simulink model "discrete_ex"  (R2024a)
settings: Solver=ode15s  StartTime=0.0  StopTime=.2  FixedStep=T/50  RelTol=1e-3
undefined symbols (not defined in the file): Down, T, Up, Vo_ref
libraries: fl_lib x10, nesl_utility x10, ee_lib x2, simulink x1, eePwmGenerator x1
settings Model: Creator=guerr  LastModifiedBy=nicholas
settings SolverCC: ZeroCrossAlgorithm=Adaptive  AlgebraicLoopSolver=LineSearch
settings DebuggingCC: IgnoredZcDiagnostic=none  UnconnectedInputMsg=warning  UnconnectedOutputMsg=warning  UnconnectedLineMsg=warning
settings ModelReferenceCC: EnableRefExpFcnMdlSchedulingChecks=on
settings SFSimCC: CustomCodeUndefinedFunction=UseInterfaceOnly
settings RTWCC: GPUComputeCapability=3.5
settings SimscapeCC: SimscapeNormalizeSystem=off

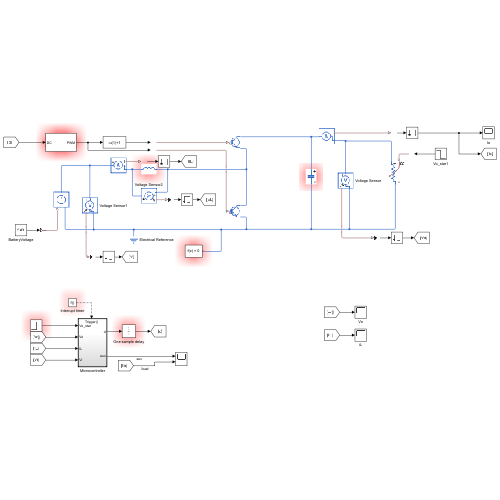
[thumbnail: Simulink's stored preview of the top-level diagram]
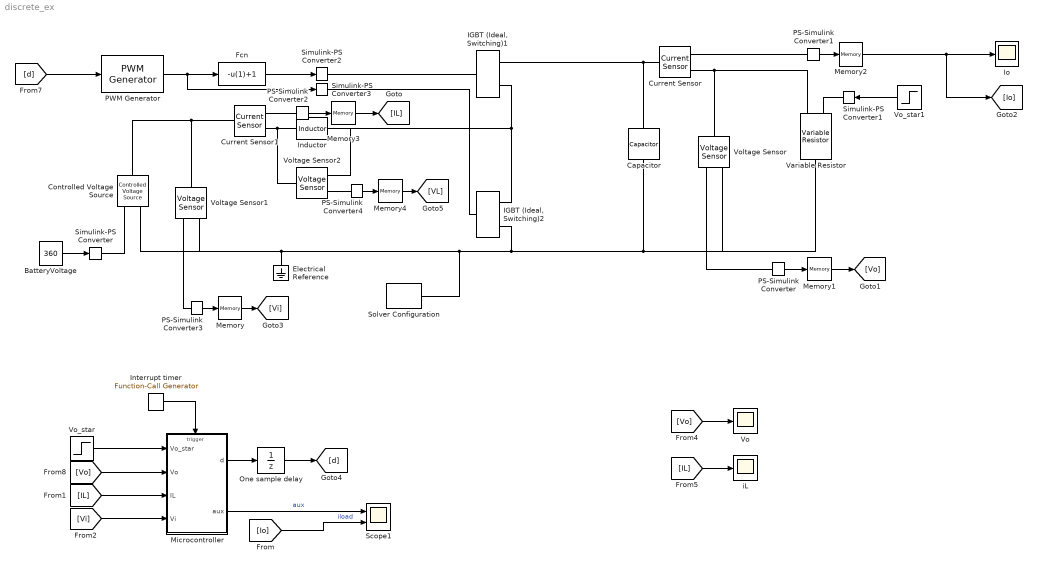
== system discrete_ex ==
  BatteryVoltage : Constant  Value=360
  Capacitor : fl_lib/Electrical/Electrical Elements/Capacitor  c=Co F  r=1.8e-3 Ohm  g=0 1/Ohm  i_specify=off  i_priority=None  i=0 A  i_nominal_specify=off  i_nominal_value=1  i_nominal_unit=A  v_specify=off  v_priority=None  v=0 V  v_nominal_specify=off  v_nominal_value=1  v_nominal_unit=V  vc_specify=on  vc_priority=High  vc=565 V  vc_nominal_specify=off  vc_nominal_value=1  vc_nominal_unit=V
  Controlled Voltage Source : fl_lib/Electrical/Electrical Sources/Controlled Voltage Source
  Current Sensor : fl_lib/Electrical/Electrical Sensors/Current Sensor
  Current Sensor1 : fl_lib/Electrical/Electrical Sensors/Current Sensor
  Electrical Reference : fl_lib/Electrical/Electrical Elements/Electrical Reference
  Fcn : Fcn  Expr=-u(1)+1
  "IGBT (Ideal, Switching)1" : ee_lib/Semiconductors & Converters/IGBT (Ideal, Switching)  port_option=ee.enum.controlport.ps  Vf=0.8 V  Ron=0.001 Ohm  Goff=1e-5 1/Ohm  Vth=.5 V  diode_param=2  diode_Vf=0.8 V  diode_Ron=0.001 Ohm  diode_Goff=1e-5 1/Ohm  diode_C=50e-9 F  diode_iRM=-235 A  diode_iF=300 A  diode_idot=-50 A/us  diode_trr_param=1  diode_trr_factor=3  diode_trr=15 us  diode_Qrr=1500 s*uA  ice_specify=off  ice_priority=None  ice=0 A  ice_nominal_specify=off  ice_nominal_value=1  ice_nominal_unit=A  vce_specify=off  vce_priority=None  vce=0 V  vce_nominal_specify=off  vce_nominal_value=1  vce_nominal_unit=V  vge_specify=off  vge_priority=None  vge=0 V  vge_nominal_specify=off  vge_nominal_value=1  vge_nominal_unit=V  thermal_loss_option=2  Von_data=[0, 1.1, 1.3, 1.45, 1.75, 2.25, 2.7; 0, 1, 1.15, 1.35, 1.7, 2.35, 3] V  Tj=[298.15, 398.15] K  Iout_data=[0, 10, 50, 100, 200, 400, 600] A  Eon_data=[0, .29, 1.43, 2.86, 5.71, 13.14, 22.86; 0, .57, 2.63, 5.14, 10.29, 20.57, 30.29] * 1e-3 J  Eoff_data=[0, .21, 1.07, 2.14, 4.29, 9.86, 17.14; 0, .43, 1.97, 3.86, 7.71, 15.43, 22.71] * 1e-3 J  Eon_data_3D=[zeros(2, 9, 3)] J  Eoff_data_3D=[zeros(2, 9, 3)] J  Tj_loss=[298.15, 398.15] K  Iout_data_loss=[0, .1, 1, 5, 10, 20, 40, 70, 100] A  tabulateWithVce=false  Vce_loss=[0, 150, 300] V  Eon_scalar=22.86e-3 J  Eoff_scalar=17.14e-3 J  Voff=300 V  Iout_scalar=600 A  useCurrentFromPreviousCycle=false  useVoltageFromPreviousCycle=false  diodeModelType=ee.enum.converters.diodeModelType.pwl  diodeTableType=ee.enum.diode.tableType.IfMat  diode_ReverseIVType=ee.enum.diode.diodeReverseIV.constant  diode_IfMat=[.07, .12, .19, 1.75, 4.24, 7.32, 11.2; .16, .3, .72, 2.14, 4.02, 6.35, 9.12] A  diode_VfMat=[.9, 1.15, 1.25, 1.5, 1.75, 2.17, 2.6, 2.85; .58, .68, .75, 1.1, 1.38, 1.77, 2.27, 2.7] V  diode_TjVec=[25, 125] degC  diode_VfVec=[.5, .7, .9, 1.3, 1.7, 2.1, 2.5] V  diode_IfVec=[.1, .2, .5, 1, 2, 4, 7, 10] A  diode_IrMat=[1e-06, 2e-06, 5e-06, 1e-05, 2.5e-05, 5e-05, .0001; 2e-06, 5e-06, 1e-05, 4e-05, 8e-05, .0002, .0005] A  diode_VrMat=[10, 100, 200, 250, 300, 325, 350; 10, 70, 160, 220, 270, 300, 320] V  diode_VrVec=[10, 20, 40, 50, 70, 80, 100] V  diode_IrVec=[1e-06, 2e-06, 5e-06, 1e-05, 2e-05, 5e-05, .0001] A  diode_Vr=-600 V  diode_Ls=150 nH  diode_Erec=0.03 J  diode_rec_loss_model=ee.enum.diode.reverseRecoveryModel.fixed  diode_ErecVal=0 J  diode_scaleWithIandV=true  diode_ErecMat=zeros(2, 3) J  diode_TjrecVec=[298.15, 398.15] K  diode_IfrecVec=[.1, 1, 10] A  diode_IrecVal=10 A  diode_VrecVal=10 V  diode_tFilter=1 / 1000 / 100 s  thermal_network_parameterization=ee.enum.thermalNetworkTopology.external  Rth=[.08, .5] K/W  Rth_Cauer=[.08, .1, .5] K/W  Rth_Foster=[.08, .14, .22, .16] K/W  thermal_mass_parameterization=ee.enum.thermalNetwork.timeconstant  thermal_mass=[.01, .5] J/K  thermal_mass_Cauer=[.01, .1, .5] J/K  thermal_mass_Foster=[.001, .005, .05, .5] J/K  thermal_time_constant=[.001, .2] s  thermal_time_constant_Cauer=[.001, .1, .2] s  thermal_time_constant_Foster=[7e-05, .0007, .01, .08] s  thermal_mass_initial_temperatures=[25, 25] degC  thermal_mass_initial_temperatures_Cauer=[25, 25, 25] degC  junction_thermal_mass=0.01 J/K  Tvec_initial_Foster=[25, 25, 25, 25] degC  no_thermal_network=0  junction_temperature_specify=off  junction_temperature_priority=None  junction_temperature=25 degC  junction_temperature_nominal_specify=off  junction_temperature_nominal_value=1  junction_temperature_nominal_unit=degC  Qj_specify=off  Qj_priority=None  Qj=0 W  Qj_nominal_specify=off  Qj_nominal_value=1  Qj_nominal_unit=W  accumulatedSwitchingLosses_specify=off  accumulatedSwitchingLosses_priority=None  accumulatedSwitchingLosses=0 J
  "IGBT (Ideal, Switching)2" : ee_lib/Semiconductors & Converters/IGBT (Ideal, Switching)  port_option=ee.enum.controlport.ps  Vf=0.8 V  Ron=0.001 Ohm  Goff=1e-5 1/Ohm  Vth=.5 V  diode_param=2  diode_Vf=0.8 V  diode_Ron=0.001 Ohm  diode_Goff=1e-5 1/Ohm  diode_C=50e-9 F  diode_iRM=-235 A  diode_iF=300 A  diode_idot=-50 A/us  diode_trr_param=1  diode_trr_factor=3  diode_trr=15 us  diode_Qrr=1500 s*uA  ice_specify=off  ice_priority=None  ice=0 A  ice_nominal_specify=off  ice_nominal_value=1  ice_nominal_unit=A  vce_specify=off  vce_priority=None  vce=0 V  vce_nominal_specify=off  vce_nominal_value=1  vce_nominal_unit=V  vge_specify=off  vge_priority=None  vge=0 V  vge_nominal_specify=off  vge_nominal_value=1  vge_nominal_unit=V  thermal_loss_option=2  Von_data=[0, 1.1, 1.3, 1.45, 1.75, 2.25, 2.7; 0, 1, 1.15, 1.35, 1.7, 2.35, 3] V  Tj=[298.15, 398.15] K  Iout_data=[0, 10, 50, 100, 200, 400, 600] A  Eon_data=[0, .29, 1.43, 2.86, 5.71, 13.14, 22.86; 0, .57, 2.63, 5.14, 10.29, 20.57, 30.29] * 1e-3 J  Eoff_data=[0, .21, 1.07, 2.14, 4.29, 9.86, 17.14; 0, .43, 1.97, 3.86, 7.71, 15.43, 22.71] * 1e-3 J  Eon_data_3D=[zeros(2, 9, 3)] J  Eoff_data_3D=[zeros(2, 9, 3)] J  Tj_loss=[298.15, 398.15] K  Iout_data_loss=[0, .1, 1, 5, 10, 20, 40, 70, 100] A  tabulateWithVce=false  Vce_loss=[0, 150, 300] V  Eon_scalar=22.86e-3 J  Eoff_scalar=17.14e-3 J  Voff=300 V  Iout_scalar=600 A  useCurrentFromPreviousCycle=false  useVoltageFromPreviousCycle=false  diodeModelType=ee.enum.converters.diodeModelType.pwl  diodeTableType=ee.enum.diode.tableType.IfMat  diode_ReverseIVType=ee.enum.diode.diodeReverseIV.constant  diode_IfMat=[.07, .12, .19, 1.75, 4.24, 7.32, 11.2; .16, .3, .72, 2.14, 4.02, 6.35, 9.12] A  diode_VfMat=[.9, 1.15, 1.25, 1.5, 1.75, 2.17, 2.6, 2.85; .58, .68, .75, 1.1, 1.38, 1.77, 2.27, 2.7] V  diode_TjVec=[25, 125] degC  diode_VfVec=[.5, .7, .9, 1.3, 1.7, 2.1, 2.5] V  diode_IfVec=[.1, .2, .5, 1, 2, 4, 7, 10] A  diode_IrMat=[1e-06, 2e-06, 5e-06, 1e-05, 2.5e-05, 5e-05, .0001; 2e-06, 5e-06, 1e-05, 4e-05, 8e-05, .0002, .0005] A  diode_VrMat=[10, 100, 200, 250, 300, 325, 350; 10, 70, 160, 220, 270, 300, 320] V  diode_VrVec=[10, 20, 40, 50, 70, 80, 100] V  diode_IrVec=[1e-06, 2e-06, 5e-06, 1e-05, 2e-05, 5e-05, .0001] A  diode_Vr=-600 V  diode_Ls=150 nH  diode_Erec=0.03 J  diode_rec_loss_model=ee.enum.diode.reverseRecoveryModel.fixed  diode_ErecVal=0 J  diode_scaleWithIandV=true  diode_ErecMat=zeros(2, 3) J  diode_TjrecVec=[298.15, 398.15] K  diode_IfrecVec=[.1, 1, 10] A  diode_IrecVal=10 A  diode_VrecVal=10 V  diode_tFilter=1 / 1000 / 100 s  thermal_network_parameterization=ee.enum.thermalNetworkTopology.external  Rth=[.08, .5] K/W  Rth_Cauer=[.08, .1, .5] K/W  Rth_Foster=[.08, .14, .22, .16] K/W  thermal_mass_parameterization=ee.enum.thermalNetwork.timeconstant  thermal_mass=[.01, .5] J/K  thermal_mass_Cauer=[.01, .1, .5] J/K  thermal_mass_Foster=[.001, .005, .05, .5] J/K  thermal_time_constant=[.001, .2] s  thermal_time_constant_Cauer=[.001, .1, .2] s  thermal_time_constant_Foster=[7e-05, .0007, .01, .08] s  thermal_mass_initial_temperatures=[25, 25] degC  thermal_mass_initial_temperatures_Cauer=[25, 25, 25] degC  junction_thermal_mass=0.01 J/K  Tvec_initial_Foster=[25, 25, 25, 25] degC  no_thermal_network=0  junction_temperature_specify=off  junction_temperature_priority=None  junction_temperature=25 degC  junction_temperature_nominal_specify=off  junction_temperature_nominal_value=1  junction_temperature_nominal_unit=degC  Qj_specify=off  Qj_priority=None  Qj=0 W  Qj_nominal_specify=off  Qj_nominal_value=1  Qj_nominal_unit=W  accumulatedSwitchingLosses_specify=off  accumulatedSwitchingLosses_priority=None  accumulatedSwitchingLosses=0 J
  Inductor : fl_lib/Electrical/Electrical Elements/Inductor  l=L H  r=R Ohm  g=1e-9 1/Ohm  i_specify=off  i_priority=None  i=0 A  i_nominal_specify=off  i_nominal_value=1  i_nominal_unit=A  v_specify=off  v_priority=None  v=0 V  v_nominal_specify=off  v_nominal_value=1  v_nominal_unit=V  i_L_specify=off  i_L_priority=High  i_L=0 A  i_L_nominal_specify=off  i_L_nominal_value=1  i_L_nominal_unit=A
  Interrupt timer : simulink/Ports & Subsystems/Function-Call Generator  sample_time=T  numberOfIterations=1  DisallowWideOutput=off
  Io : Scope
  Memory{,1..4} (5 alike) : Memory
  Microcontroller : Subsystem
  One sample delay : UnitDelay  SampleTime=T  HasFrameUpgradeWarning=on
  PS-Simulink Converter{,1..4} (5 alike) : nesl_utility/PS-Simulink Converter  PhysicalDomain=network_engine_domain  SubClassName=ps_output  LeftPortType=input  RightPortType=output  PseudoPeriodic=off  Frequencies=[]  VectorFormat=1-D array  Unit=1  AffineConversion=off
  PWM Generator : eePwmGenerator/PWM Generator  CarrCount=Up-Down  Tper=T/2  Tdelay=0  Ts=T/100
  Scope1 : Scope  NumInputPorts=2
  Simulink-PS Converter{,1..3} (4 alike) : nesl_utility/Simulink-PS Converter  PhysicalDomain=network_engine_domain  SubClassName=ps_input  LeftPortType=input  RightPortType=output  PseudoPeriodic=off  Frequencies=[]  NoiseDistribution=none  NoiseParameters=[]  Unit=1  AffineConversion=off  FilteringAndDerivatives=provide  SimscapeFilterOrder=1  InputFilterTimeConstant=0.001  UdotUserProvided=0
  Solver Configuration : nesl_utility/Solver Configuration  PhysicalDomain=network_engine_domain  SubClassName=solver  LeftPortType=input  RightPortType=generic  Tones=[]  Harmonics=[]  SimulateNoise=off  Profile=off  UseLocalSampling=off  EnableSwitchedLinearOptims=on  FrequencyDomain=off  UseCCode=off  RelTol=0.001  AbsTol=1e-06  MinStep=1e-09  ToWorkspace=off  RevertToSquareIcSolve=off  NumHomotopyIterations=100  PhasorMode=off  PhasorModeNumHarmonics=1  ConsistencySolver=NEWTON_FTOL  IndexReductionMethod=DerivativeReplacement  DoDC=off  ResidualTolerance=1e-09  ConsistencyTolSource=GLOBAL  ConsistencyAbsTol=0.001  ConsistencyRelTol=0.001  ConsistencyTolFactor=0.001  UseLocalSolver=on  LocalSolverChoice=NE_TRAPEZOIDAL_ADVANCER  ResolveIndetEquations=on  FunctionEvalNumThread=1  LocalSolverSampleTime=T/100  DoFixedCost=on  MaxNonlinIter=3  MaxModeIter=2  ComputeImpulses=off  ImpulseIterations=2  LinearAlgebra=auto  LinearAlgebraNumThread=0  EquationFormulation=NE_TIME_EF  DelaysMemoryBudget=1024  AutomaticFiltering=on  FilteringTimeConstant=0.001  PartitionStorageMethod=AS_NEEDED  PartitionMemoryBudget=1024  PartitionMethod=ROBUST  MultibodyUseLocalSolver=off  MultibodyLocalSolverChoice=ODE1  MultibodyLocalSolverSampleTime=0.001
  Variable Resistor : fl_lib/Electrical/Electrical Elements/Variable Resistor  Rmin=565/100 Ohm  thermalEnable=false  thermal_mass=1 J/K  i_specify=off  i_priority=None  i=0 A  i_nominal_specify=off  i_nominal_value=1  i_nominal_unit=A  v_specify=on  v_priority=Low  v=565 V  v_nominal_specify=off  v_nominal_value=1  v_nominal_unit=V  T_specify=off  T_priority=None  T=300 K  T_nominal_specify=off  T_nominal_value=1  T_nominal_unit=K
  Vo : Scope
  Vo_star : Step  Time=0  After=Vo_ref  SampleTime=0
  Vo_star1 : Step  Time=.1  Before=565/55  After=565/90  SampleTime=0
  Voltage Sensor : fl_lib/Electrical/Electrical Sensors/Voltage Sensor
  Voltage Sensor1 : fl_lib/Electrical/Electrical Sensors/Voltage Sensor
  Voltage Sensor2 : fl_lib/Electrical/Electrical Sensors/Voltage Sensor
  iL : Scope
  wires:
  BatteryVoltage/1 -> Simulink-PS Converter/1
  [d] -> PWM Generator/1
  PWM Generator/1 -> Simulink-PS Converter3/1, Fcn/1
  Fcn/1 -> Simulink-PS Converter2/1
  PS-Simulink Converter2/1 -> Memory3/1
  PS-Simulink Converter3/1 -> Memory/1
  PS-Simulink Converter1/1 -> Memory2/1
  PS-Simulink Converter/1 -> Memory1/1
  PS-Simulink Converter4/1 -> Memory4/1
  Memory/1 -> [Vi]
  Memory2/1 -> [Io], Io/1
  Memory1/1 -> [Vo]
  Memory3/1 -> [IL]
  Memory4/1 -> [VL]
  Vo_star1/1 -> Simulink-PS Converter1/1
  Interrupt timer/1 -> Microcontroller/Trigger
  [Io] -> Scope1/2  "iload"
  [Vo] -> Microcontroller/2("Vo ")
  Microcontroller/1(d) -> One sample delay/1
  [IL] -> Microcontroller/3(IL)
  Microcontroller/2(aux) -> Scope1/1  "aux"
  Vo_star/1 -> Microcontroller/1(Vo_star)
  One sample delay/1 -> [d]
  [Vi] -> Microcontroller/4(Vi)
  [Vo] -> Vo/1
  [IL] -> iL/1
  connections:
  Capacitor/RConn1 -- Variable Resistor/RConn1 -- Voltage Sensor/RConn2 -- Solver Configuration/RConn1 -- Voltage Sensor1/RConn2 -- Controlled Voltage Source/RConn2 -- Electrical Reference/LConn1 -- "IGBT (Ideal, Switching)2"/RConn2
  Simulink-PS Converter/RConn1 -- Controlled Voltage Source/RConn1
  Current Sensor/RConn2 -- Variable Resistor/LConn2 -- Voltage Sensor/LConn1
  Simulink-PS Converter2/RConn1 -- "IGBT (Ideal, Switching)1"/LConn1
  Simulink-PS Converter3/RConn1 -- "IGBT (Ideal, Switching)2"/LConn1
  PS-Simulink Converter/LConn1 -- Voltage Sensor/RConn1
  Capacitor/LConn1 -- "IGBT (Ideal, Switching)1"/RConn1 -- Current Sensor/LConn1
  PS-Simulink Converter1/LConn1 -- Current Sensor/RConn1
  Current Sensor1/LConn1 -- Voltage Sensor1/LConn1 -- Controlled Voltage Source/LConn1
  Current Sensor1/RConn2 -- Voltage Sensor2/LConn1 -- Inductor/LConn1
  PS-Simulink Converter2/LConn1 -- Current Sensor1/RConn1
  Voltage Sensor1/RConn1 -- PS-Simulink Converter3/LConn1
  "IGBT (Ideal, Switching)1"/RConn2 -- "IGBT (Ideal, Switching)2"/RConn1 -- Voltage Sensor2/RConn2 -- Inductor/RConn1
  Voltage Sensor2/RConn1 -- PS-Simulink Converter4/LConn1
  Simulink-PS Converter1/RConn1 -- Variable Resistor/LConn1

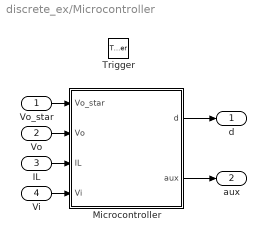
== system discrete_ex/Microcontroller ==
  Vo_star : Inport
  "Vo " : Inport  Port=2
  IL : Inport  Port=3
  Vi : Inport  Port=4
  Trigger : TriggerPort  TriggerType=function-call  VariantControl=Variant
  Microcontroller : MATLAB Function  TreatAsAtomicUnit=on
  d : Outport  VectorParamsAs1DForOutWhenUnconnected=off
  aux : Outport  Port=2  VectorParamsAs1DForOutWhenUnconnected=off
  wires:
  Vi/1 -> Microcontroller/4(Vi)
  "Vo "/1 -> Microcontroller/2(Vo)
  Microcontroller/1(d) -> d/1
  Vo_star/1 -> Microcontroller/1(Vo_star)
  IL/1 -> Microcontroller/3(IL)
  Microcontroller/2(aux) -> aux/1

== matlab function discrete_ex/Microcontroller/Microcontroller ==
  data: Vo_star input; Vo input; IL input; d output; Vi input; aux output
function [d,aux] = microcontroller(Vo_star,Vo,IL,Vi)


% Declare your constants below
% Boost converter
fc = 20000; % (Hz) Switching frequency
T = 1/fc; % (s) sampling period
L = 5e-3; % (H)
R = 0.14; % (Ohm)
Co = 1186.5e-6; % (F) 
I_max = 250; % (A) Nissan leaf drive max current

% Current controller params
% Zero-pole cancellation
bw = 250; % (Hz) Closed-loop bandwidth
kp = 2*pi*bw*L;
ki = 2*pi*bw*R; % zero-pole cancellation - (maybe poor distrubance rejection)

% Maximum overshoot (neglecting zero - might require prefilter)
% Mp = .10; % (p.u.) Overshoot
% wn = 2*pi*bw; % (rad/s) Natural frequency
% theta = atan(-pi/log(Mp));
% xi = cos(theta);
% kp = 2*xi*wn*L-R;
% ki = wn^2*L;

% Voltage controller params
bw = 25; % (Hz) closed-loop bandwidth

%Only P
% kp_v = 2*pi*bw*Co;
% ki_v = 0;

% PI controller
% Option 1 - Free selection of parameters
% Mp = .1; % (p.u.)  overshoot
% wn = 2*pi*bw; % (rad/s) Natural frequency (approx bandwidth)
% theta = atan(-pi/log(Mp));
% xi = cos(theta);
% kp_v = 2*xi*wn*Co;
% ki_v = wn^2*Co;

% Option 2 - A maximum kp gain is required
kp_v = 2*pi*bw*Co; % As taken for P controller or any other value
Mp = .1; % (p.u.)  overshoot
theta = atan(-pi/log(Mp));
xi = cos(theta);
wn = kp_v/(2*xi*Co); % (rad/s) Natural frequency
ki_v = wn^2*Co;


% Declare your variables below
% Current controller variables
persistent io_star_k;
persistent io_star_k_1;
persistent eil_k;
persistent eil_k_1

% Voltage controller variables
persistent vl_star_k;
persistent vl_star_k_1;
persistent evo_k;
persistent evo_k_1;
persistent il_star_k;


% Initialize your variables
if isempty(vl_star_k)
    vl_star_k = 0;
    vl_star_k_1 = 0;
    eil_k = 0;
    eil_k_1 = 0;
    io_star_k = 0;
    io_star_k_1 = 0;
    evo_k = 0;
    evo_k_1 = 0;
    il_star_k = 0;
end

% Execute your algorithm
% Voltage controller
evo_k = Vo_star - Vo;
io_star_k = io_star_k_1 + (T/2*ki_v+kp_v)*evo_k + (T/2*ki_v-kp_v)*evo_k_1;

% Convert (approximate to steady-state value) into boost current
gain = (Vi- R*il_star_k)/(Vo_star);
il_star_k = io_star_k/gain;

% Check current limits & realizable references calculation
if (il_star_k > I_max)
    il_star_k = I_max;
    evo_k = evo_k + 1/(T/2*ki_v+kp_v)*(il_star_k*gain - io_star_k);
    io_star_k = il_star_k*gain;
end

if (il_star_k < -I_max)
    il_star_k = -I_max;
    evo_k = evo_k + 1/(T/2*ki_v+kp_v)*(il_star_k*gain - io_star_k);
    io_star_k = il_star_k*gain;
end

% Current controller
eil_k = il_star_k - IL;
vl_star_k = vl_star_k_1 + (T/2*ki+kp)*eil_k + (T/2*ki-kp)*eil_k_1;

% Check voltage limits & realizable references calculation
% Including previous controller
if (vl_star_k > Vi/2)   % Limit to Vi/2 to allow continous power transfer
    eil_k = eil_k + 1/(T/2*ki+kp)*(Vi/2 - vl_star_k);
    vl_star_k = Vi/2;
    il_star_k = IL+eil_k; % Calculate boost current realizable reference
    evo_k = evo_k + 1/(T/2*ki_v+kp_v)*(il_star_k*gain - io_star_k);
    io_star_k = il_star_k*gain;
end

if (vl_star_k < (Vi - Vo))   % Limit to Vi/2 to allow continous power transfer
    eil_k = eil_k + 1/(T/2*ki+kp)*((Vi - Vo) - vl_star_k);
    vl_star_k = (Vi - Vo);
    il_star_k = IL+eil_k; % Calculate boost current realizable reference
    evo_k = evo_k + 1/(T/2*ki_v+kp_v)*(il_star_k*gain - io_star_k);
    io_star_k = il_star_k*gain;
end


% Calculate duty
d = min([1 max([0 1 + (vl_star_k - Vi)/Vo])]);

aux = io_star_k;
% Update variables
io_star_k_1 = io_star_k;
eil_k_1 = eil_k;
vl_star_k_1 = vl_star_k;
evo_k_1 = evo_k;
